simulink subsystem "ControlAdapter"  (R2022b)
settings: Solver=VariableStepAuto  StartTime=0.0  StopTime=10.0  RelTol=1e-3
settings Model: Creator=ycheb  LastModifiedBy=ycheb
settings OptimizationCC: ReuseModelBlockBuffer=on

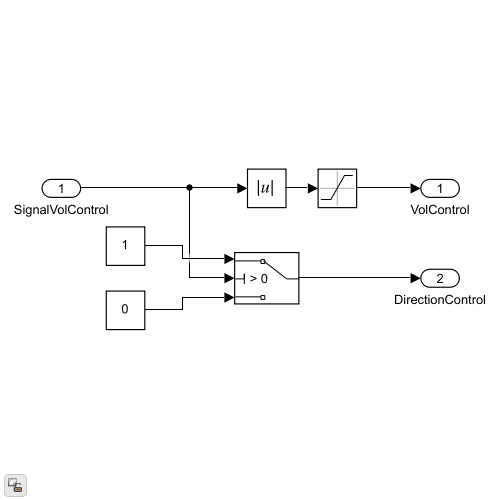
[thumbnail: Simulink's stored preview of the top-level diagram]
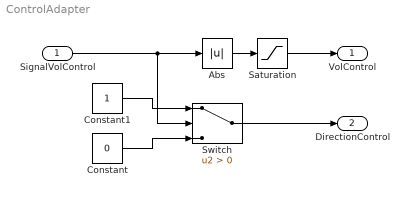
== system ControlAdapter ==
  SignalVolControl : Inport
  Abs : Abs  SaturateOnIntegerOverflow=off
  Constant : Constant  Value=0  OutDataTypeStr=boolean
  Constant1 : Constant  OutDataTypeStr=boolean
  Saturation : Saturate  UpperLimit=3.3  LowerLimit=0
  Switch : Switch  Criteria=u2 > Threshold  SaturateOnIntegerOverflow=off  InputSameDT=off
  VolControl : Outport
  DirectionControl : Outport  Port=2  OutDataTypeStr=boolean
  wires:
  Constant/1 -> Switch/3
  Saturation/1 -> VolControl/1
  Abs/1 -> Saturation/1
  Constant1/1 -> Switch/1
  SignalVolControl/1 -> Abs/1, Switch/2
  Switch/1 -> DirectionControl/1
